simulink model "gs_pid_closed_loop"  (R2024b)
settings: Solver=ode45  StartTime=0.0  StopTime=2  MaxStep=0.001  RelTol=1e-3
model workspace (MAT data in the model file):
  Gs_den = [1 7.2 144]
  Gs_num = 144
  Kd = 0.1834
  Ki = 21.002
  Kp = 4.5122
  Tf = 0.01
settings Model: Creator=santi  LastModifiedBy=santi

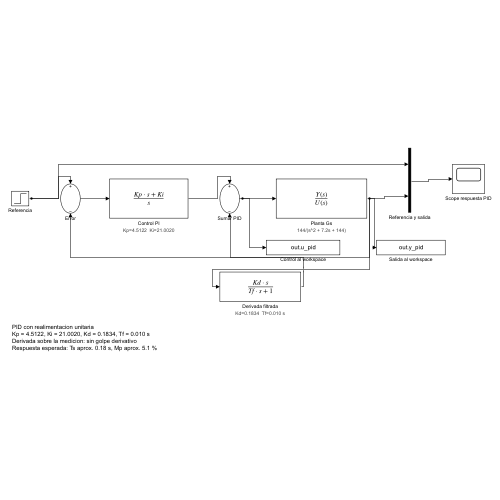
[thumbnail: Simulink's stored preview of the top-level diagram]
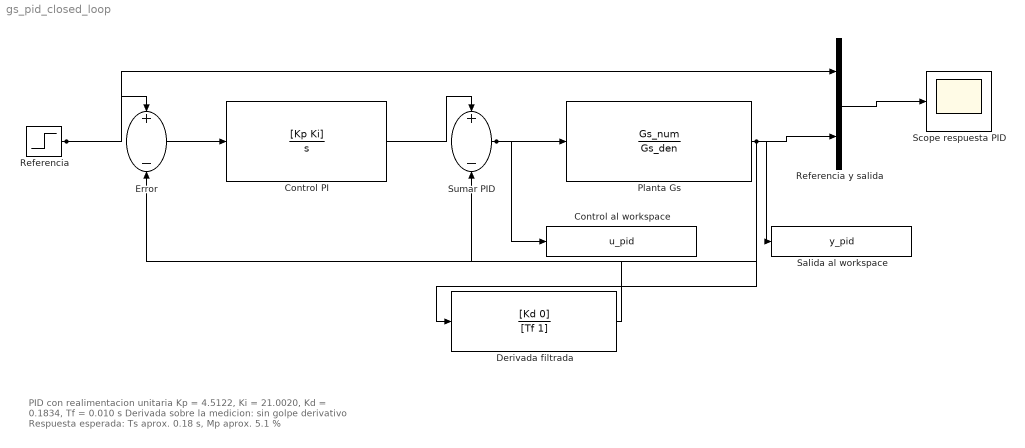
== system gs_pid_closed_loop ==
  note: PID con realimentacion unitaria
      | Kp = 4.5122, Ki = 21.0020, Kd = 0.1834, Tf = 0.010 s
      | Derivada sobre la medicion: sin golpe derivativo
      | Respuesta esperada: Ts aprox. 0.18 s, Mp aprox. 5.1 %
  Control PI : TransferFcn  Numerator=[Kp Ki]  Denominator=[1 0]
      settings: AttributesFormatString="Kp=4.5122  Ki=21.0020"
  Control al workspace : ToWorkspace  VariableName=u_pid  SaveFormat=Structure With Time  SampleTime=-1
  Derivada filtrada : TransferFcn  Numerator=[Kd 0]  Denominator=[Tf 1]
      settings: AttributesFormatString="Kd=0.1834  Tf=0.010 s"
  Error : Sum  Inputs=+-
  Planta Gs : TransferFcn  Numerator=Gs_num  Denominator=Gs_den
      settings: AttributesFormatString=144/(s^2 + 7.2s + 144)
  Referencia : Step  Time=0.1  SampleTime=0
  Referencia y salida : Mux  Inputs=2
  Salida al workspace : ToWorkspace  VariableName=y_pid  SaveFormat=Structure With Time  SampleTime=-1
  Scope respuesta PID : Scope
  Sumar PID : Sum  Inputs=+-
  wires:
  Referencia/1 -> Error/1, Referencia y salida/1
  Error/1 -> Control PI/1
  Control PI/1 -> Sumar PID/1
  Sumar PID/1 -> Planta Gs/1, Control al workspace/1
  Planta Gs/1 -> Error/2, Derivada filtrada/1, Referencia y salida/2, Salida al workspace/1
  Derivada filtrada/1 -> Sumar PID/2
  Referencia y salida/1 -> Scope respuesta PID/1
